simulink model "c00010M_harness"  (R2018a)
settings: Solver=FixedStepAuto  StartTime=0.0  StopTime=300  FixedStep=0.1  RelTol=1e-3
undefined symbols (not defined in the file): A1, hmax, PriorityTank, R1, R2, sigbuilder_block, TempThreshold
(part 29 of 40)

== system c00010M_harness/M119/Tank2/Control/ManualControlLiquidInOut ==
  Fill : Inport
  Empty : Inport  Port=2
  LiquidLevel : Inport  Port=3
  Constant : Constant  Value=hmax*0.9
  Constant1 : Constant  Value=0.9
  Logical Operator{,1..2,4} (4 alike) : Logic  AllPortsSameDT=off  OutDataTypeStr=boolean
  Logical Operator3 : Logic  Operator=NOT  AllPortsSameDT=off  OutDataTypeStr=boolean
  Logical Operator5 : Logic  Operator=NOT  AllPortsSameDT=off  OutDataTypeStr=boolean
  Relational Operator1 : RelationalOperator  Operator=<  OutDataTypeStr=boolean  RndMeth=Simplest
  Relational Operator2 : RelationalOperator  Operator=<  OutDataTypeStr=boolean  RndMeth=Simplest
  LiquidIn : Outport
  LiquidOut : Outport  Port=2
  wires:
  Empty/1 -> Logical Operator1/2
  Constant/1 -> Relational Operator1/2
  Relational Operator1/1 -> Logical Operator/2
  Fill/1 -> Logical Operator/1
  Logical Operator/1 -> Logical Operator5/1, Logical Operator2/1
  Relational Operator2/1 -> Logical Operator1/1
  Logical Operator1/1 -> Logical Operator3/1, Logical Operator4/2
  Constant1/1 -> Relational Operator2/1
  LiquidLevel/1 -> Relational Operator2/2, Relational Operator1/1
  Logical Operator3/1 -> Logical Operator2/2
  Logical Operator2/1 -> LiquidIn/1
  Logical Operator5/1 -> Logical Operator4/1
  Logical Operator4/1 -> LiquidOut/1

== system c00010M_harness/M119/Tank3/Control/Maintenance ==
  Type : Inport
  StartMaintenance : Inport  Port=2
  LiquidLevel : Inport  Port=3
  Chart : Stateflow chart  TreatAsAtomicUnit=on
  LiquidIn : Outport
  LiquidOut : Outport  Port=2
  wires:
  StartMaintenance/1 -> Chart/2(StartMaintenance)
  Type/1 -> Chart/1(Type)
  LiquidLevel/1 -> Chart/3(LiquidLevel)
  Chart/1(LiquidIn) -> LiquidIn/1
  Chart/2(LiquidOut) -> LiquidOut/1

== system c00010M_harness/M119/Tank3/Control/ManualControlLiquidInOut ==
  Fill : Inport
  Empty : Inport  Port=2
  LiquidLevel : Inport  Port=3
  Constant : Constant  Value=hmax*0.9
  Constant1 : Constant  Value=0.001
  Logical Operator{,1..2,4} (4 alike) : Logic  AllPortsSameDT=off  OutDataTypeStr=boolean
  Logical Operator3 : Logic  Operator=NOT  AllPortsSameDT=off  OutDataTypeStr=boolean
  Logical Operator5 : Logic  Operator=NOT  AllPortsSameDT=off  OutDataTypeStr=boolean
  Relational Operator1 : RelationalOperator  Operator=<  OutDataTypeStr=boolean  RndMeth=Simplest
  Relational Operator2 : RelationalOperator  Operator=<  OutDataTypeStr=boolean  RndMeth=Simplest
  LiquidIn : Outport
  LiquidOut : Outport  Port=2
  wires:
  Empty/1 -> Logical Operator1/2
  Constant/1 -> Relational Operator1/2
  Relational Operator1/1 -> Logical Operator/2
  Fill/1 -> Logical Operator/1
  Logical Operator/1 -> Logical Operator5/1, Logical Operator2/1
  Relational Operator2/1 -> Logical Operator1/1
  Logical Operator1/1 -> Logical Operator3/1, Logical Operator4/2
  Constant1/1 -> Relational Operator2/1
  LiquidLevel/1 -> Relational Operator2/2, Relational Operator1/1
  Logical Operator3/1 -> Logical Operator2/2
  Logical Operator2/1 -> LiquidIn/1
  Logical Operator5/1 -> Logical Operator4/1
  Logical Operator4/1 -> LiquidOut/1

== system c00010M_harness/M119/Tank3/Control/ManualControlReference ==
  ManualReference : Inport
  LiquidLevel : Inport  Port=2
  Add : Sum  Inputs=+-
  Add1 : Sum  Inputs=+-
  Gain1 : Gain  Gain=0.95
  Gain2 : Gain  Gain=0.95
  Relational Operator : RelationalOperator  Operator=>  OutDataTypeStr=boolean  RndMeth=Simplest
  Relational Operator1 : RelationalOperator  Operator=<  OutDataTypeStr=boolean  RndMeth=Simplest
  Saturation1 : Saturate  UpperLimit=hmax*0.9  LowerLimit=0
  LiquidIn : Outport
  LiquidOut : Outport  Port=2
  wires:
  LiquidLevel/1 -> Relational Operator/2, Add/1, Add1/1, Gain2/1
  Relational Operator/1 -> LiquidIn/1
  Relational Operator1/1 -> LiquidOut/1
  Add/1 -> Add1/2
  Add1/1 -> Relational Operator1/2
  Gain1/1 -> Saturation1/1
  Gain2/1 -> Add/2
  ManualReference/1 -> Gain1/1
  Saturation1/1 -> Relational Operator1/1, Relational Operator/1

== system c00010M_harness/M120/Tank2/Control/ManualControlLiquidInOut ==
  Fill : Inport
  Empty : Inport  Port=2
  LiquidLevel : Inport  Port=3
  Constant : Constant  Value=hmax*0.9
  Constant1 : Constant  Value=0.001
  Logical Operator : Logic  Operator=OR  AllPortsSameDT=off  OutDataTypeStr=boolean
  Logical Operator1 : Logic  AllPortsSameDT=off  OutDataTypeStr=boolean
  Logical Operator2 : Logic  AllPortsSameDT=off  OutDataTypeStr=boolean
  Logical Operator3 : Logic  Operator=NOT  AllPortsSameDT=off  OutDataTypeStr=boolean
  Logical Operator4 : Logic  AllPortsSameDT=off  OutDataTypeStr=boolean
  Logical Operator5 : Logic  Operator=NOT  AllPortsSameDT=off  OutDataTypeStr=boolean
  Relational Operator1 : RelationalOperator  Operator=<  OutDataTypeStr=boolean  RndMeth=Simplest
  Relational Operator2 : RelationalOperator  Operator=<  OutDataTypeStr=boolean  RndMeth=Simplest
  LiquidIn : Outport
  LiquidOut : Outport  Port=2
  wires:
  Empty/1 -> Logical Operator1/2
  Constant/1 -> Relational Operator1/2
  Relational Operator1/1 -> Logical Operator/2
  Fill/1 -> Logical Operator/1
  Logical Operator/1 -> Logical Operator5/1, Logical Operator2/1
  Relational Operator2/1 -> Logical Operator1/1
  Logical Operator1/1 -> Logical Operator3/1, Logical Operator4/2
  Constant1/1 -> Relational Operator2/1
  LiquidLevel/1 -> Relational Operator2/2, Relational Operator1/1
  Logical Operator3/1 -> Logical Operator2/2
  Logical Operator2/1 -> LiquidIn/1
  Logical Operator5/1 -> Logical Operator4/1
  Logical Operator4/1 -> LiquidOut/1

== system c00010M_harness/M120/Tank3/Control/Maintenance ==
  Type : Inport
  StartMaintenance : Inport  Port=2
  LiquidLevel : Inport  Port=3
  Chart : Stateflow chart  TreatAsAtomicUnit=on
  LiquidIn : Outport
  LiquidOut : Outport  Port=2
  wires:
  StartMaintenance/1 -> Chart/2(StartMaintenance)
  Type/1 -> Chart/1(Type)
  LiquidLevel/1 -> Chart/3(LiquidLevel)
  Chart/1(LiquidIn) -> LiquidIn/1
  Chart/2(LiquidOut) -> LiquidOut/1

== system c00010M_harness/M120/Tank3/Control/ManualControlLiquidInOut ==
  Fill : Inport
  Empty : Inport  Port=2
  LiquidLevel : Inport  Port=3
  Constant : Constant  Value=hmax*0.9
  Constant1 : Constant  Value=0.001
  Logical Operator{,1..2,4} (4 alike) : Logic  AllPortsSameDT=off  OutDataTypeStr=boolean
  Logical Operator3 : Logic  Operator=NOT  AllPortsSameDT=off  OutDataTypeStr=boolean
  Logical Operator5 : Logic  Operator=NOT  AllPortsSameDT=off  OutDataTypeStr=boolean
  Relational Operator1 : RelationalOperator  Operator=<  OutDataTypeStr=boolean  RndMeth=Simplest
  Relational Operator2 : RelationalOperator  Operator=<  OutDataTypeStr=boolean  RndMeth=Simplest
  LiquidIn : Outport
  LiquidOut : Outport  Port=2
  wires:
  Empty/1 -> Logical Operator1/2
  Constant/1 -> Relational Operator1/2
  Relational Operator1/1 -> Logical Operator/2
  Fill/1 -> Logical Operator/1
  Logical Operator/1 -> Logical Operator5/1, Logical Operator2/1
  Relational Operator2/1 -> Logical Operator1/1
  Logical Operator1/1 -> Logical Operator3/1, Logical Operator4/2
  Constant1/1 -> Relational Operator2/1
  LiquidLevel/1 -> Relational Operator2/2, Relational Operator1/1
  Logical Operator3/1 -> Logical Operator2/2
  Logical Operator2/1 -> LiquidIn/1
  Logical Operator5/1 -> Logical Operator4/1
  Logical Operator4/1 -> LiquidOut/1

== system c00010M_harness/M120/Tank3/Control/ManualControlReference ==
  ManualReference : Inport
  LiquidLevel : Inport  Port=2
  Add : Sum  Inputs=+-
  Add1 : Sum  Inputs=+-
  Gain1 : Gain  Gain=0.95
  Gain2 : Gain  Gain=0.95
  Relational Operator : RelationalOperator  Operator=>  OutDataTypeStr=boolean  RndMeth=Simplest
  Relational Operator1 : RelationalOperator  Operator=<  OutDataTypeStr=boolean  RndMeth=Simplest
  Saturation1 : Saturate  UpperLimit=hmax*0.9  LowerLimit=0
  LiquidIn : Outport
  LiquidOut : Outport  Port=2
  wires:
  LiquidLevel/1 -> Relational Operator/2, Add/1, Add1/1, Gain2/1
  Relational Operator/1 -> LiquidIn/1
  Relational Operator1/1 -> LiquidOut/1
  Add/1 -> Add1/2
  Add1/1 -> Relational Operator1/2
  Gain1/1 -> Saturation1/1
  Gain2/1 -> Add/2
  ManualReference/1 -> Gain1/1
  Saturation1/1 -> Relational Operator1/1, Relational Operator/1

== system c00010M_harness/M121/Tank2/Control/ManualControlLiquidInOut ==
  Fill : Inport
  Empty : Inport  Port=2
  LiquidLevel : Inport  Port=3
  Constant : Constant  Value=hmax*0.9
  Constant1 : Constant  Value=0.001
  Logical Operator : Logic  AllPortsSameDT=off  OutDataTypeStr=boolean
  Logical Operator1 : Logic  Operator=OR  AllPortsSameDT=off  OutDataTypeStr=boolean
  Logical Operator2 : Logic  AllPortsSameDT=off  OutDataTypeStr=boolean
  Logical Operator3 : Logic  Operator=NOT  AllPortsSameDT=off  OutDataTypeStr=boolean
  Logical Operator4 : Logic  AllPortsSameDT=off  OutDataTypeStr=boolean
  Logical Operator5 : Logic  Operator=NOT  AllPortsSameDT=off  OutDataTypeStr=boolean
  Relational Operator1 : RelationalOperator  Operator=<  OutDataTypeStr=boolean  RndMeth=Simplest
  Relational Operator2 : RelationalOperator  Operator=<  OutDataTypeStr=boolean  RndMeth=Simplest
  LiquidIn : Outport
  LiquidOut : Outport  Port=2
  wires:
  Empty/1 -> Logical Operator1/2
  Constant/1 -> Relational Operator1/2
  Relational Operator1/1 -> Logical Operator/2
  Fill/1 -> Logical Operator/1
  Logical Operator/1 -> Logical Operator5/1, Logical Operator2/1
  Relational Operator2/1 -> Logical Operator1/1
  Logical Operator1/1 -> Logical Operator3/1, Logical Operator4/2
  Constant1/1 -> Relational Operator2/1
  LiquidLevel/1 -> Relational Operator2/2, Relational Operator1/1
  Logical Operator3/1 -> Logical Operator2/2
  Logical Operator2/1 -> LiquidIn/1
  Logical Operator5/1 -> Logical Operator4/1
  Logical Operator4/1 -> LiquidOut/1

== system c00010M_harness/M121/Tank3/Control/Maintenance ==
  Type : Inport
  StartMaintenance : Inport  Port=2
  LiquidLevel : Inport  Port=3
  Chart : Stateflow chart  TreatAsAtomicUnit=on
  LiquidIn : Outport
  LiquidOut : Outport  Port=2
  wires:
  StartMaintenance/1 -> Chart/2(StartMaintenance)
  Type/1 -> Chart/1(Type)
  LiquidLevel/1 -> Chart/3(LiquidLevel)
  Chart/1(LiquidIn) -> LiquidIn/1
  Chart/2(LiquidOut) -> LiquidOut/1

== system c00010M_harness/M121/Tank3/Control/ManualControlLiquidInOut ==
  Fill : Inport
  Empty : Inport  Port=2
  LiquidLevel : Inport  Port=3
  Constant : Constant  Value=hmax*0.9
  Constant1 : Constant  Value=0.001
  Logical Operator{,1..2,4} (4 alike) : Logic  AllPortsSameDT=off  OutDataTypeStr=boolean
  Logical Operator3 : Logic  Operator=NOT  AllPortsSameDT=off  OutDataTypeStr=boolean
  Logical Operator5 : Logic  Operator=NOT  AllPortsSameDT=off  OutDataTypeStr=boolean
  Relational Operator1 : RelationalOperator  Operator=<  OutDataTypeStr=boolean  RndMeth=Simplest
  Relational Operator2 : RelationalOperator  Operator=<  OutDataTypeStr=boolean  RndMeth=Simplest
  LiquidIn : Outport
  LiquidOut : Outport  Port=2
  wires:
  Empty/1 -> Logical Operator1/2
  Constant/1 -> Relational Operator1/2
  Relational Operator1/1 -> Logical Operator/2
  Fill/1 -> Logical Operator/1
  Logical Operator/1 -> Logical Operator5/1, Logical Operator2/1
  Relational Operator2/1 -> Logical Operator1/1
  Logical Operator1/1 -> Logical Operator3/1, Logical Operator4/2
  Constant1/1 -> Relational Operator2/1
  LiquidLevel/1 -> Relational Operator2/2, Relational Operator1/1
  Logical Operator3/1 -> Logical Operator2/2
  Logical Operator2/1 -> LiquidIn/1
  Logical Operator5/1 -> Logical Operator4/1
  Logical Operator4/1 -> LiquidOut/1

== system c00010M_harness/M121/Tank3/Control/ManualControlReference ==
  ManualReference : Inport
  LiquidLevel : Inport  Port=2
  Add : Sum  Inputs=+-
  Add1 : Sum  Inputs=+-
  Gain1 : Gain  Gain=0.95
  Gain2 : Gain  Gain=0.95
  Relational Operator : RelationalOperator  Operator=>  OutDataTypeStr=boolean  RndMeth=Simplest
  Relational Operator1 : RelationalOperator  Operator=<  OutDataTypeStr=boolean  RndMeth=Simplest
  Saturation1 : Saturate  UpperLimit=hmax*0.9  LowerLimit=0
  LiquidIn : Outport
  LiquidOut : Outport  Port=2
  wires:
  LiquidLevel/1 -> Relational Operator/2, Add/1, Add1/1, Gain2/1
  Relational Operator/1 -> LiquidIn/1
  Relational Operator1/1 -> LiquidOut/1
  Add/1 -> Add1/2
  Add1/1 -> Relational Operator1/2
  Gain1/1 -> Saturation1/1
  Gain2/1 -> Add/2
  ManualReference/1 -> Gain1/1
  Saturation1/1 -> Relational Operator1/1, Relational Operator/1

== system c00010M_harness/M122/Tank2/Control/ManualControlLiquidInOut ==
  Fill : Inport
  Empty : Inport  Port=2
  LiquidLevel : Inport  Port=3
  Constant : Constant  Value=hmax*0.9
  Constant1 : Constant  Value=0.001
  Logical Operator : Logic  AllPortsSameDT=off  OutDataTypeStr=boolean
  Logical Operator1 : Logic  AllPortsSameDT=off  OutDataTypeStr=boolean
  Logical Operator2 : Logic  Operator=OR  AllPortsSameDT=off  OutDataTypeStr=boolean
  Logical Operator3 : Logic  Operator=NOT  AllPortsSameDT=off  OutDataTypeStr=boolean
  Logical Operator4 : Logic  AllPortsSameDT=off  OutDataTypeStr=boolean
  Logical Operator5 : Logic  Operator=NOT  AllPortsSameDT=off  OutDataTypeStr=boolean
  Relational Operator1 : RelationalOperator  Operator=<  OutDataTypeStr=boolean  RndMeth=Simplest
  Relational Operator2 : RelationalOperator  Operator=<  OutDataTypeStr=boolean  RndMeth=Simplest
  LiquidIn : Outport
  LiquidOut : Outport  Port=2
  wires:
  Empty/1 -> Logical Operator1/2
  Constant/1 -> Relational Operator1/2
  Relational Operator1/1 -> Logical Operator/2
  Fill/1 -> Logical Operator/1
  Logical Operator/1 -> Logical Operator5/1, Logical Operator2/1
  Relational Operator2/1 -> Logical Operator1/1
  Logical Operator1/1 -> Logical Operator3/1, Logical Operator4/2
  Constant1/1 -> Relational Operator2/1
  LiquidLevel/1 -> Relational Operator2/2, Relational Operator1/1
  Logical Operator3/1 -> Logical Operator2/2
  Logical Operator2/1 -> LiquidIn/1
  Logical Operator5/1 -> Logical Operator4/1
  Logical Operator4/1 -> LiquidOut/1

== system c00010M_harness/M122/Tank3/Control/Maintenance ==
  Type : Inport
  StartMaintenance : Inport  Port=2
  LiquidLevel : Inport  Port=3
  Chart : Stateflow chart  TreatAsAtomicUnit=on
  LiquidIn : Outport
  LiquidOut : Outport  Port=2
  wires:
  StartMaintenance/1 -> Chart/2(StartMaintenance)
  Type/1 -> Chart/1(Type)
  LiquidLevel/1 -> Chart/3(LiquidLevel)
  Chart/1(LiquidIn) -> LiquidIn/1
  Chart/2(LiquidOut) -> LiquidOut/1

== system c00010M_harness/M122/Tank3/Control/ManualControlLiquidInOut ==
  Fill : Inport
  Empty : Inport  Port=2
  LiquidLevel : Inport  Port=3
  Constant : Constant  Value=hmax*0.9
  Constant1 : Constant  Value=0.001
  Logical Operator{,1..2,4} (4 alike) : Logic  AllPortsSameDT=off  OutDataTypeStr=boolean
  Logical Operator3 : Logic  Operator=NOT  AllPortsSameDT=off  OutDataTypeStr=boolean
  Logical Operator5 : Logic  Operator=NOT  AllPortsSameDT=off  OutDataTypeStr=boolean
  Relational Operator1 : RelationalOperator  Operator=<  OutDataTypeStr=boolean  RndMeth=Simplest
  Relational Operator2 : RelationalOperator  Operator=<  OutDataTypeStr=boolean  RndMeth=Simplest
  LiquidIn : Outport
  LiquidOut : Outport  Port=2
  wires:
  Empty/1 -> Logical Operator1/2
  Constant/1 -> Relational Operator1/2
  Relational Operator1/1 -> Logical Operator/2
  Fill/1 -> Logical Operator/1
  Logical Operator/1 -> Logical Operator5/1, Logical Operator2/1
  Relational Operator2/1 -> Logical Operator1/1
  Logical Operator1/1 -> Logical Operator3/1, Logical Operator4/2
  Constant1/1 -> Relational Operator2/1
  LiquidLevel/1 -> Relational Operator2/2, Relational Operator1/1
  Logical Operator3/1 -> Logical Operator2/2
  Logical Operator2/1 -> LiquidIn/1
  Logical Operator5/1 -> Logical Operator4/1
  Logical Operator4/1 -> LiquidOut/1

== system c00010M_harness/M122/Tank3/Control/ManualControlReference ==
  ManualReference : Inport
  LiquidLevel : Inport  Port=2
  Add : Sum  Inputs=+-
  Add1 : Sum  Inputs=+-
  Gain1 : Gain  Gain=0.95
  Gain2 : Gain  Gain=0.95
  Relational Operator : RelationalOperator  Operator=>  OutDataTypeStr=boolean  RndMeth=Simplest
  Relational Operator1 : RelationalOperator  Operator=<  OutDataTypeStr=boolean  RndMeth=Simplest
  Saturation1 : Saturate  UpperLimit=hmax*0.9  LowerLimit=0
  LiquidIn : Outport
  LiquidOut : Outport  Port=2
  wires:
  LiquidLevel/1 -> Relational Operator/2, Add/1, Add1/1, Gain2/1
  Relational Operator/1 -> LiquidIn/1
  Relational Operator1/1 -> LiquidOut/1
  Add/1 -> Add1/2
  Add1/1 -> Relational Operator1/2
  Gain1/1 -> Saturation1/1
  Gain2/1 -> Add/2
  ManualReference/1 -> Gain1/1
  Saturation1/1 -> Relational Operator1/1, Relational Operator/1

== system c00010M_harness/M123/Tank2/Control/ManualControlLiquidInOut ==
  Fill : Inport
  Empty : Inport  Port=2
  LiquidLevel : Inport  Port=3
  Constant : Constant  Value=hmax*0.9
  Constant1 : Constant  Value=0.001
  Logical Operator{,1..2,4} (4 alike) : Logic  AllPortsSameDT=off  OutDataTypeStr=boolean
  Logical Operator5 : Logic  Operator=NOT  AllPortsSameDT=off  OutDataTypeStr=boolean
  Relational Operator1 : RelationalOperator  Operator=<  OutDataTypeStr=boolean  RndMeth=Simplest
  Relational Operator2 : RelationalOperator  Operator=<  OutDataTypeStr=boolean  RndMeth=Simplest
  LiquidIn : Outport
  LiquidOut : Outport  Port=2
  wires:
  Empty/1 -> Logical Operator1/2
  Constant/1 -> Relational Operator1/2
  Relational Operator1/1 -> Logical Operator/2
  Fill/1 -> Logical Operator/1
  Logical Operator/1 -> Logical Operator5/1, Logical Operator2/1
  Relational Operator2/1 -> Logical Operator1/1
  Constant1/1 -> Relational Operator2/1
  LiquidLevel/1 -> Relational Operator2/2, Relational Operator1/1
  Logical Operator1/1 -> Logical Operator2/2, Logical Operator4/2
  Logical Operator2/1 -> LiquidIn/1
  Logical Operator5/1 -> Logical Operator4/1
  Logical Operator4/1 -> LiquidOut/1

== system c00010M_harness/M123/Tank3/Control/Maintenance ==
  Type : Inport
  StartMaintenance : Inport  Port=2
  LiquidLevel : Inport  Port=3
  Chart : Stateflow chart  TreatAsAtomicUnit=on
  LiquidIn : Outport
  LiquidOut : Outport  Port=2
  wires:
  StartMaintenance/1 -> Chart/2(StartMaintenance)
  Type/1 -> Chart/1(Type)
  LiquidLevel/1 -> Chart/3(LiquidLevel)
  Chart/1(LiquidIn) -> LiquidIn/1
  Chart/2(LiquidOut) -> LiquidOut/1

== system c00010M_harness/M123/Tank3/Control/ManualControlLiquidInOut ==
  Fill : Inport
  Empty : Inport  Port=2
  LiquidLevel : Inport  Port=3
  Constant : Constant  Value=hmax*0.9
  Constant1 : Constant  Value=0.001
  Logical Operator{,1..2,4} (4 alike) : Logic  AllPortsSameDT=off  OutDataTypeStr=boolean
  Logical Operator3 : Logic  Operator=NOT  AllPortsSameDT=off  OutDataTypeStr=boolean
  Logical Operator5 : Logic  Operator=NOT  AllPortsSameDT=off  OutDataTypeStr=boolean
  Relational Operator1 : RelationalOperator  Operator=<  OutDataTypeStr=boolean  RndMeth=Simplest
  Relational Operator2 : RelationalOperator  Operator=<  OutDataTypeStr=boolean  RndMeth=Simplest
  LiquidIn : Outport
  LiquidOut : Outport  Port=2
  wires:
  Empty/1 -> Logical Operator1/2
  Constant/1 -> Relational Operator1/2
  Relational Operator1/1 -> Logical Operator/2
  Fill/1 -> Logical Operator/1
  Logical Operator/1 -> Logical Operator5/1, Logical Operator2/1
  Relational Operator2/1 -> Logical Operator1/1
  Logical Operator1/1 -> Logical Operator3/1, Logical Operator4/2
  Constant1/1 -> Relational Operator2/1
  LiquidLevel/1 -> Relational Operator2/2, Relational Operator1/1
  Logical Operator3/1 -> Logical Operator2/2
  Logical Operator2/1 -> LiquidIn/1
  Logical Operator5/1 -> Logical Operator4/1
  Logical Operator4/1 -> LiquidOut/1

== system c00010M_harness/M123/Tank3/Control/ManualControlReference ==
  ManualReference : Inport
  LiquidLevel : Inport  Port=2
  Add : Sum  Inputs=+-
  Add1 : Sum  Inputs=+-
  Gain1 : Gain  Gain=0.95
  Gain2 : Gain  Gain=0.95
  Relational Operator : RelationalOperator  Operator=>  OutDataTypeStr=boolean  RndMeth=Simplest
  Relational Operator1 : RelationalOperator  Operator=<  OutDataTypeStr=boolean  RndMeth=Simplest
  Saturation1 : Saturate  UpperLimit=hmax*0.9  LowerLimit=0
  LiquidIn : Outport
  LiquidOut : Outport  Port=2
  wires:
  LiquidLevel/1 -> Relational Operator/2, Add/1, Add1/1, Gain2/1
  Relational Operator/1 -> LiquidIn/1
  Relational Operator1/1 -> LiquidOut/1
  Add/1 -> Add1/2
  Add1/1 -> Relational Operator1/2
  Gain1/1 -> Saturation1/1
  Gain2/1 -> Add/2
  ManualReference/1 -> Gain1/1
  Saturation1/1 -> Relational Operator1/1, Relational Operator/1

== system c00010M_harness/M124/Tank2/Control/ManualControlLiquidInOut ==
  Fill : Inport
  Empty : Inport  Port=2
  LiquidLevel : Inport  Port=3
  Constant : Constant  Value=hmax*0.9
  Constant1 : Constant  Value=0.001
  Logical Operator : Logic  AllPortsSameDT=off  OutDataTypeStr=boolean
  Logical Operator1 : Logic  AllPortsSameDT=off  OutDataTypeStr=boolean
  Logical Operator2 : Logic  AllPortsSameDT=off  OutDataTypeStr=boolean
  Logical Operator3 : Logic  Operator=NOT  AllPortsSameDT=off  OutDataTypeStr=boolean
  Logical Operator4 : Logic  Operator=OR  AllPortsSameDT=off  OutDataTypeStr=boolean
  Logical Operator5 : Logic  Operator=NOT  AllPortsSameDT=off  OutDataTypeStr=boolean
  Relational Operator1 : RelationalOperator  Operator=<  OutDataTypeStr=boolean  RndMeth=Simplest
  Relational Operator2 : RelationalOperator  Operator=<  OutDataTypeStr=boolean  RndMeth=Simplest
  LiquidIn : Outport
  LiquidOut : Outport  Port=2
  wires:
  Empty/1 -> Logical Operator1/2
  Constant/1 -> Relational Operator1/2
  Relational Operator1/1 -> Logical Operator/2
  Fill/1 -> Logical Operator/1
  Logical Operator/1 -> Logical Operator5/1, Logical Operator2/1
  Relational Operator2/1 -> Logical Operator1/1
  Logical Operator1/1 -> Logical Operator3/1, Logical Operator4/2
  Constant1/1 -> Relational Operator2/1
  LiquidLevel/1 -> Relational Operator2/2, Relational Operator1/1
  Logical Operator3/1 -> Logical Operator2/2
  Logical Operator2/1 -> LiquidIn/1
  Logical Operator5/1 -> Logical Operator4/1
  Logical Operator4/1 -> LiquidOut/1

== system c00010M_harness/M124/Tank3/Control/Maintenance ==
  Type : Inport
  StartMaintenance : Inport  Port=2
  LiquidLevel : Inport  Port=3
  Chart : Stateflow chart  TreatAsAtomicUnit=on
  LiquidIn : Outport
  LiquidOut : Outport  Port=2
  wires:
  StartMaintenance/1 -> Chart/2(StartMaintenance)
  Type/1 -> Chart/1(Type)
  LiquidLevel/1 -> Chart/3(LiquidLevel)
  Chart/1(LiquidIn) -> LiquidIn/1
  Chart/2(LiquidOut) -> LiquidOut/1

== system c00010M_harness/M124/Tank3/Control/ManualControlLiquidInOut ==
  Fill : Inport
  Empty : Inport  Port=2
  LiquidLevel : Inport  Port=3
  Constant : Constant  Value=hmax*0.9
  Constant1 : Constant  Value=0.001
  Logical Operator{,1..2,4} (4 alike) : Logic  AllPortsSameDT=off  OutDataTypeStr=boolean
  Logical Operator3 : Logic  Operator=NOT  AllPortsSameDT=off  OutDataTypeStr=boolean
  Logical Operator5 : Logic  Operator=NOT  AllPortsSameDT=off  OutDataTypeStr=boolean
  Relational Operator1 : RelationalOperator  Operator=<  OutDataTypeStr=boolean  RndMeth=Simplest
  Relational Operator2 : RelationalOperator  Operator=<  OutDataTypeStr=boolean  RndMeth=Simplest
  LiquidIn : Outport
  LiquidOut : Outport  Port=2
  wires:
  Empty/1 -> Logical Operator1/2
  Constant/1 -> Relational Operator1/2
  Relational Operator1/1 -> Logical Operator/2
  Fill/1 -> Logical Operator/1
  Logical Operator/1 -> Logical Operator5/1, Logical Operator2/1
  Relational Operator2/1 -> Logical Operator1/1
  Logical Operator1/1 -> Logical Operator3/1, Logical Operator4/2
  Constant1/1 -> Relational Operator2/1
  LiquidLevel/1 -> Relational Operator2/2, Relational Operator1/1
  Logical Operator3/1 -> Logical Operator2/2
  Logical Operator2/1 -> LiquidIn/1
  Logical Operator5/1 -> Logical Operator4/1
  Logical Operator4/1 -> LiquidOut/1

== system c00010M_harness/M124/Tank3/Control/ManualControlReference ==
  ManualReference : Inport
  LiquidLevel : Inport  Port=2
  Add : Sum  Inputs=+-
  Add1 : Sum  Inputs=+-
  Gain1 : Gain  Gain=0.95
  Gain2 : Gain  Gain=0.95
  Relational Operator : RelationalOperator  Operator=>  OutDataTypeStr=boolean  RndMeth=Simplest
  Relational Operator1 : RelationalOperator  Operator=<  OutDataTypeStr=boolean  RndMeth=Simplest
  Saturation1 : Saturate  UpperLimit=hmax*0.9  LowerLimit=0
  LiquidIn : Outport
  LiquidOut : Outport  Port=2
  wires:
  LiquidLevel/1 -> Relational Operator/2, Add/1, Add1/1, Gain2/1
  Relational Operator/1 -> LiquidIn/1
  Relational Operator1/1 -> LiquidOut/1
  Add/1 -> Add1/2
  Add1/1 -> Relational Operator1/2
  Gain1/1 -> Saturation1/1
  Gain2/1 -> Add/2
  ManualReference/1 -> Gain1/1
  Saturation1/1 -> Relational Operator1/1, Relational Operator/1

== system c00010M_harness/M125/Tank2/Control/ManualControlLiquidInOut ==
  Fill : Inport
  Empty : Inport  Port=2
  LiquidLevel : Inport  Port=3
  Constant : Constant  Value=hmax*0.9
  Constant1 : Constant  Value=0.001
  Logical Operator{,1..2,4} (4 alike) : Logic  AllPortsSameDT=off  OutDataTypeStr=boolean
  Logical Operator3 : Logic  Operator=NOT  AllPortsSameDT=off  OutDataTypeStr=boolean
  Relational Operator1 : RelationalOperator  Operator=<  OutDataTypeStr=boolean  RndMeth=Simplest
  Relational Operator2 : RelationalOperator  Operator=<  OutDataTypeStr=boolean  RndMeth=Simplest
  LiquidIn : Outport
  LiquidOut : Outport  Port=2
  wires:
  Empty/1 -> Logical Operator1/2
  Constant/1 -> Relational Operator1/2
  Relational Operator1/1 -> Logical Operator/2
  Fill/1 -> Logical Operator/1
  Relational Operator2/1 -> Logical Operator1/1
  Logical Operator1/1 -> Logical Operator3/1, Logical Operator4/2
  Constant1/1 -> Relational Operator2/1
  LiquidLevel/1 -> Relational Operator2/2, Relational Operator1/1
  Logical Operator3/1 -> Logical Operator2/2
  Logical Operator2/1 -> LiquidIn/1
  Logical Operator/1 -> Logical Operator4/1, Logical Operator2/1
  Logical Operator4/1 -> LiquidOut/1

== system c00010M_harness/M125/Tank3/Control/Maintenance ==
  Type : Inport
  StartMaintenance : Inport  Port=2
  LiquidLevel : Inport  Port=3
  Chart : Stateflow chart  TreatAsAtomicUnit=on
  LiquidIn : Outport
  LiquidOut : Outport  Port=2
  wires:
  StartMaintenance/1 -> Chart/2(StartMaintenance)
  Type/1 -> Chart/1(Type)
  LiquidLevel/1 -> Chart/3(LiquidLevel)
  Chart/1(LiquidIn) -> LiquidIn/1
  Chart/2(LiquidOut) -> LiquidOut/1

== system c00010M_harness/M125/Tank3/Control/ManualControlLiquidInOut ==
  Fill : Inport
  Empty : Inport  Port=2
  LiquidLevel : Inport  Port=3
  Constant : Constant  Value=hmax*0.9
  Constant1 : Constant  Value=0.001
  Logical Operator{,1..2,4} (4 alike) : Logic  AllPortsSameDT=off  OutDataTypeStr=boolean
  Logical Operator3 : Logic  Operator=NOT  AllPortsSameDT=off  OutDataTypeStr=boolean
  Logical Operator5 : Logic  Operator=NOT  AllPortsSameDT=off  OutDataTypeStr=boolean
  Relational Operator1 : RelationalOperator  Operator=<  OutDataTypeStr=boolean  RndMeth=Simplest
  Relational Operator2 : RelationalOperator  Operator=<  OutDataTypeStr=boolean  RndMeth=Simplest
  LiquidIn : Outport
  LiquidOut : Outport  Port=2
  wires:
  Empty/1 -> Logical Operator1/2
  Constant/1 -> Relational Operator1/2
  Relational Operator1/1 -> Logical Operator/2
  Fill/1 -> Logical Operator/1
  Logical Operator/1 -> Logical Operator5/1, Logical Operator2/1
  Relational Operator2/1 -> Logical Operator1/1
  Logical Operator1/1 -> Logical Operator3/1, Logical Operator4/2
  Constant1/1 -> Relational Operator2/1
  LiquidLevel/1 -> Relational Operator2/2, Relational Operator1/1
  Logical Operator3/1 -> Logical Operator2/2
  Logical Operator2/1 -> LiquidIn/1
  Logical Operator5/1 -> Logical Operator4/1
  Logical Operator4/1 -> LiquidOut/1

== system c00010M_harness/M125/Tank3/Control/ManualControlReference ==
  ManualReference : Inport
  LiquidLevel : Inport  Port=2
  Add : Sum  Inputs=+-
  Add1 : Sum  Inputs=+-
  Gain1 : Gain  Gain=0.95
  Gain2 : Gain  Gain=0.95
  Relational Operator : RelationalOperator  Operator=>  OutDataTypeStr=boolean  RndMeth=Simplest
  Relational Operator1 : RelationalOperator  Operator=<  OutDataTypeStr=boolean  RndMeth=Simplest
  Saturation1 : Saturate  UpperLimit=hmax*0.9  LowerLimit=0
  LiquidIn : Outport
  LiquidOut : Outport  Port=2
  wires:
  LiquidLevel/1 -> Relational Operator/2, Add/1, Add1/1, Gain2/1
  Relational Operator/1 -> LiquidIn/1
  Relational Operator1/1 -> LiquidOut/1
  Add/1 -> Add1/2
  Add1/1 -> Relational Operator1/2
  Gain1/1 -> Saturation1/1
  Gain2/1 -> Add/2
  ManualReference/1 -> Gain1/1
  Saturation1/1 -> Relational Operator1/1, Relational Operator/1

== system c00010M_harness/M126/Tank2/Control/ManualControlLiquidInOut ==
  Fill : Inport
  Empty : Inport  Port=2
  LiquidLevel : Inport  Port=3
  Constant : Constant  Value=hmax*0.9
  Constant1 : Constant  Value=0.001
  Logical Operator{,1..2,4} (4 alike) : Logic  AllPortsSameDT=off  OutDataTypeStr=boolean
  Logical Operator3 : Logic  Operator=NOT  AllPortsSameDT=off  OutDataTypeStr=boolean
  Logical Operator5 : Logic  Operator=NOT  AllPortsSameDT=off  OutDataTypeStr=boolean
  Relational Operator1 : RelationalOperator  Operator=>  OutDataTypeStr=boolean  RndMeth=Simplest
  Relational Operator2 : RelationalOperator  Operator=<  OutDataTypeStr=boolean  RndMeth=Simplest
  LiquidIn : Outport
  LiquidOut : Outport  Port=2
  wires:
  Empty/1 -> Logical Operator1/2
  Constant/1 -> Relational Operator1/2
  Relational Operator1/1 -> Logical Operator/2
  Fill/1 -> Logical Operator/1
  Logical Operator/1 -> Logical Operator5/1, Logical Operator2/1
  Relational Operator2/1 -> Logical Operator1/1
  Logical Operator1/1 -> Logical Operator3/1, Logical Operator4/2
  Constant1/1 -> Relational Operator2/1
  LiquidLevel/1 -> Relational Operator2/2, Relational Operator1/1
  Logical Operator3/1 -> Logical Operator2/2
  Logical Operator2/1 -> LiquidIn/1
  Logical Operator5/1 -> Logical Operator4/1
  Logical Operator4/1 -> LiquidOut/1

== system c00010M_harness/M126/Tank3/Control/Maintenance ==
  Type : Inport
  StartMaintenance : Inport  Port=2
  LiquidLevel : Inport  Port=3
  Chart : Stateflow chart  TreatAsAtomicUnit=on
  LiquidIn : Outport
  LiquidOut : Outport  Port=2
  wires:
  StartMaintenance/1 -> Chart/2(StartMaintenance)
  Type/1 -> Chart/1(Type)
  LiquidLevel/1 -> Chart/3(LiquidLevel)
  Chart/1(LiquidIn) -> LiquidIn/1
  Chart/2(LiquidOut) -> LiquidOut/1

== system c00010M_harness/M126/Tank3/Control/ManualControlLiquidInOut ==
  Fill : Inport
  Empty : Inport  Port=2
  LiquidLevel : Inport  Port=3
  Constant : Constant  Value=hmax*0.9
  Constant1 : Constant  Value=0.001
  Logical Operator{,1..2,4} (4 alike) : Logic  AllPortsSameDT=off  OutDataTypeStr=boolean
  Logical Operator3 : Logic  Operator=NOT  AllPortsSameDT=off  OutDataTypeStr=boolean
  Logical Operator5 : Logic  Operator=NOT  AllPortsSameDT=off  OutDataTypeStr=boolean
  Relational Operator1 : RelationalOperator  Operator=<  OutDataTypeStr=boolean  RndMeth=Simplest
  Relational Operator2 : RelationalOperator  Operator=<  OutDataTypeStr=boolean  RndMeth=Simplest
  LiquidIn : Outport
  LiquidOut : Outport  Port=2
  wires:
  Empty/1 -> Logical Operator1/2
  Constant/1 -> Relational Operator1/2
  Relational Operator1/1 -> Logical Operator/2
  Fill/1 -> Logical Operator/1
  Logical Operator/1 -> Logical Operator5/1, Logical Operator2/1
  Relational Operator2/1 -> Logical Operator1/1
  Logical Operator1/1 -> Logical Operator3/1, Logical Operator4/2
  Constant1/1 -> Relational Operator2/1
  LiquidLevel/1 -> Relational Operator2/2, Relational Operator1/1
  Logical Operator3/1 -> Logical Operator2/2
  Logical Operator2/1 -> LiquidIn/1
  Logical Operator5/1 -> Logical Operator4/1
  Logical Operator4/1 -> LiquidOut/1

== system c00010M_harness/M126/Tank3/Control/ManualControlReference ==
  ManualReference : Inport
  LiquidLevel : Inport  Port=2
  Add : Sum  Inputs=+-
  Add1 : Sum  Inputs=+-
  Gain1 : Gain  Gain=0.95
  Gain2 : Gain  Gain=0.95
  Relational Operator : RelationalOperator  Operator=>  OutDataTypeStr=boolean  RndMeth=Simplest
  Relational Operator1 : RelationalOperator  Operator=<  OutDataTypeStr=boolean  RndMeth=Simplest
  Saturation1 : Saturate  UpperLimit=hmax*0.9  LowerLimit=0
  LiquidIn : Outport
  LiquidOut : Outport  Port=2
  wires:
  LiquidLevel/1 -> Relational Operator/2, Add/1, Add1/1, Gain2/1
  Relational Operator/1 -> LiquidIn/1
  Relational Operator1/1 -> LiquidOut/1
  Add/1 -> Add1/2
  Add1/1 -> Relational Operator1/2
  Gain1/1 -> Saturation1/1
  Gain2/1 -> Add/2
  ManualReference/1 -> Gain1/1
  Saturation1/1 -> Relational Operator1/1, Relational Operator/1

== system c00010M_harness/M127/Tank2/Control/ManualControlLiquidInOut ==
  Fill : Inport
  Empty : Inport  Port=2
  LiquidLevel : Inport  Port=3
  Constant : Constant  Value=hmax*0.9
  Constant1 : Constant  Value=0.001
  Logical Operator{,1..2,4} (4 alike) : Logic  AllPortsSameDT=off  OutDataTypeStr=boolean
  Logical Operator3 : Logic  Operator=NOT  AllPortsSameDT=off  OutDataTypeStr=boolean
  Logical Operator5 : Logic  Operator=NOT  AllPortsSameDT=off  OutDataTypeStr=boolean
  Relational Operator1 : RelationalOperator  Operator=<  OutDataTypeStr=boolean  RndMeth=Simplest
  Relational Operator2 : RelationalOperator  Operator=>  OutDataTypeStr=boolean  RndMeth=Simplest
  LiquidIn : Outport
  LiquidOut : Outport  Port=2
  wires:
  Empty/1 -> Logical Operator1/2
  Constant/1 -> Relational Operator1/2
  Relational Operator1/1 -> Logical Operator/2
  Fill/1 -> Logical Operator/1
  Logical Operator/1 -> Logical Operator5/1, Logical Operator2/1
  Relational Operator2/1 -> Logical Operator1/1
  Logical Operator1/1 -> Logical Operator3/1, Logical Operator4/2
  Constant1/1 -> Relational Operator2/1
  LiquidLevel/1 -> Relational Operator2/2, Relational Operator1/1
  Logical Operator3/1 -> Logical Operator2/2
  Logical Operator2/1 -> LiquidIn/1
  Logical Operator5/1 -> Logical Operator4/1
  Logical Operator4/1 -> LiquidOut/1

== system c00010M_harness/M127/Tank3/Control/Maintenance ==
  Type : Inport
  StartMaintenance : Inport  Port=2
  LiquidLevel : Inport  Port=3
  Chart : Stateflow chart  TreatAsAtomicUnit=on
  LiquidIn : Outport
  LiquidOut : Outport  Port=2
  wires:
  StartMaintenance/1 -> Chart/2(StartMaintenance)
  Type/1 -> Chart/1(Type)
  LiquidLevel/1 -> Chart/3(LiquidLevel)
  Chart/1(LiquidIn) -> LiquidIn/1
  Chart/2(LiquidOut) -> LiquidOut/1

== system c00010M_harness/M127/Tank3/Control/ManualControlLiquidInOut ==
  Fill : Inport
  Empty : Inport  Port=2
  LiquidLevel : Inport  Port=3
  Constant : Constant  Value=hmax*0.9
  Constant1 : Constant  Value=0.001
  Logical Operator{,1..2,4} (4 alike) : Logic  AllPortsSameDT=off  OutDataTypeStr=boolean
  Logical Operator3 : Logic  Operator=NOT  AllPortsSameDT=off  OutDataTypeStr=boolean
  Logical Operator5 : Logic  Operator=NOT  AllPortsSameDT=off  OutDataTypeStr=boolean
  Relational Operator1 : RelationalOperator  Operator=<  OutDataTypeStr=boolean  RndMeth=Simplest
  Relational Operator2 : RelationalOperator  Operator=<  OutDataTypeStr=boolean  RndMeth=Simplest
  LiquidIn : Outport
  LiquidOut : Outport  Port=2
  wires:
  Empty/1 -> Logical Operator1/2
  Constant/1 -> Relational Operator1/2
  Relational Operator1/1 -> Logical Operator/2
  Fill/1 -> Logical Operator/1
  Logical Operator/1 -> Logical Operator5/1, Logical Operator2/1
  Relational Operator2/1 -> Logical Operator1/1
  Logical Operator1/1 -> Logical Operator3/1, Logical Operator4/2
  Constant1/1 -> Relational Operator2/1
  LiquidLevel/1 -> Relational Operator2/2, Relational Operator1/1
  Logical Operator3/1 -> Logical Operator2/2
  Logical Operator2/1 -> LiquidIn/1
  Logical Operator5/1 -> Logical Operator4/1
  Logical Operator4/1 -> LiquidOut/1

== system c00010M_harness/M127/Tank3/Control/ManualControlReference ==
  ManualReference : Inport
  LiquidLevel : Inport  Port=2
  Add : Sum  Inputs=+-
  Add1 : Sum  Inputs=+-
  Gain1 : Gain  Gain=0.95
  Gain2 : Gain  Gain=0.95
  Relational Operator : RelationalOperator  Operator=>  OutDataTypeStr=boolean  RndMeth=Simplest
  Relational Operator1 : RelationalOperator  Operator=<  OutDataTypeStr=boolean  RndMeth=Simplest
  Saturation1 : Saturate  UpperLimit=hmax*0.9  LowerLimit=0
  LiquidIn : Outport
  LiquidOut : Outport  Port=2
  wires:
  LiquidLevel/1 -> Relational Operator/2, Add/1, Add1/1, Gain2/1
  Relational Operator/1 -> LiquidIn/1
  Relational Operator1/1 -> LiquidOut/1
  Add/1 -> Add1/2
  Add1/1 -> Relational Operator1/2
  Gain1/1 -> Saturation1/1
  Gain2/1 -> Add/2
  ManualReference/1 -> Gain1/1
  Saturation1/1 -> Relational Operator1/1, Relational Operator/1

== system c00010M_harness/M139/Tank2/Control/ManualControlLiquidInOut ==
  Fill : Inport
  Empty : Inport  Port=2
  LiquidLevel : Inport  Port=3
  Constant : Constant  Value=hmax*0.9
  Constant1 : Constant  Value=0.001
  Logical Operator{,1..2,4} (4 alike) : Logic  AllPortsSameDT=off  OutDataTypeStr=boolean
  Logical Operator3 : Logic  Operator=NOT  AllPortsSameDT=off  OutDataTypeStr=boolean
  Logical Operator5 : Logic  Operator=NOT  AllPortsSameDT=off  OutDataTypeStr=boolean
  Relational Operator1 : RelationalOperator  Operator=<  OutDataTypeStr=boolean  RndMeth=Simplest
  Relational Operator2 : RelationalOperator  Operator=<  OutDataTypeStr=boolean  RndMeth=Simplest
  LiquidIn : Outport
  LiquidOut : Outport  Port=2
  wires:
  Empty/1 -> Logical Operator1/2
  Constant/1 -> Relational Operator1/2
  Relational Operator1/1 -> Logical Operator/2
  Fill/1 -> Logical Operator/1
  Logical Operator/1 -> Logical Operator5/1, Logical Operator2/1
  Relational Operator2/1 -> Logical Operator1/1
  Logical Operator1/1 -> Logical Operator3/1, Logical Operator4/2
  Constant1/1 -> Relational Operator2/1
  LiquidLevel/1 -> Relational Operator2/2, Relational Operator1/1
  Logical Operator3/1 -> Logical Operator2/2
  Logical Operator2/1 -> LiquidIn/1
  Logical Operator5/1 -> Logical Operator4/1
  Logical Operator4/1 -> LiquidOut/1

== system c00010M_harness/M139/Tank3/Control/Maintenance ==
  Type : Inport
  StartMaintenance : Inport  Port=2
  LiquidLevel : Inport  Port=3
  Chart : Stateflow chart  TreatAsAtomicUnit=on
  LiquidIn : Outport
  LiquidOut : Outport  Port=2
  wires:
  StartMaintenance/1 -> Chart/2(StartMaintenance)
  Type/1 -> Chart/1(Type)
  LiquidLevel/1 -> Chart/3(LiquidLevel)
  Chart/1(LiquidIn) -> LiquidIn/1
  Chart/2(LiquidOut) -> LiquidOut/1

== system c00010M_harness/M139/Tank3/Control/ManualControlLiquidInOut ==
  Fill : Inport
  Empty : Inport  Port=2
  LiquidLevel : Inport  Port=3
  Constant : Constant  Value=hmax*0.9
  Constant1 : Constant  Value=0.001
  Logical Operator{,1..2,4} (4 alike) : Logic  AllPortsSameDT=off  OutDataTypeStr=boolean
  Logical Operator3 : Logic  Operator=NOT  AllPortsSameDT=off  OutDataTypeStr=boolean
  Logical Operator5 : Logic  Operator=NOT  AllPortsSameDT=off  OutDataTypeStr=boolean
  Relational Operator1 : RelationalOperator  Operator=<  OutDataTypeStr=boolean  RndMeth=Simplest
  Relational Operator2 : RelationalOperator  Operator=<  OutDataTypeStr=boolean  RndMeth=Simplest
  LiquidIn : Outport
  LiquidOut : Outport  Port=2
  wires:
  Empty/1 -> Logical Operator1/2
  Constant/1 -> Relational Operator1/2
  Relational Operator1/1 -> Logical Operator/2
  Fill/1 -> Logical Operator/1
  Logical Operator/1 -> Logical Operator5/1, Logical Operator2/1
  Relational Operator2/1 -> Logical Operator1/1
  Logical Operator1/1 -> Logical Operator3/1, Logical Operator4/2
  Constant1/1 -> Relational Operator2/1
  LiquidLevel/1 -> Relational Operator2/2, Relational Operator1/1
  Logical Operator3/1 -> Logical Operator2/2
  Logical Operator2/1 -> LiquidIn/1
  Logical Operator5/1 -> Logical Operator4/1
  Logical Operator4/1 -> LiquidOut/1

== system c00010M_harness/M139/Tank3/Control/ManualControlReference ==
  ManualReference : Inport
  LiquidLevel : Inport  Port=2
  Add : Sum  Inputs=+-
  Add1 : Sum  Inputs=+-
  Gain1 : Gain  Gain=0.95
  Gain2 : Gain  Gain=0.95
  Relational Operator : RelationalOperator  Operator=>  OutDataTypeStr=boolean  RndMeth=Simplest
  Relational Operator1 : RelationalOperator  Operator=<  OutDataTypeStr=boolean  RndMeth=Simplest
  Saturation1 : Saturate  UpperLimit=hmax*0.9  LowerLimit=0
  LiquidIn : Outport
  LiquidOut : Outport  Port=2
  wires:
  LiquidLevel/1 -> Relational Operator/2, Add/1, Add1/1, Gain2/1
  Relational Operator/1 -> LiquidIn/1
  Relational Operator1/1 -> LiquidOut/1
  Add/1 -> Add1/2
  Add1/1 -> Relational Operator1/2
  Gain1/1 -> Saturation1/1
  Gain2/1 -> Add/2
  ManualReference/1 -> Gain1/1
  Saturation1/1 -> Relational Operator1/1, Relational Operator/1

== system c00010M_harness/M140/Tank2/Control/ManualControlLiquidInOut ==
  Fill : Inport
  Empty : Inport  Port=2
  LiquidLevel : Inport  Port=3
  Constant : Constant  Value=hmax*0.9
  Constant1 : Constant  Value=0.001
  Logical Operator{,1..2,4} (4 alike) : Logic  AllPortsSameDT=off  OutDataTypeStr=boolean
  Logical Operator3 : Logic  Operator=NOT  AllPortsSameDT=off  OutDataTypeStr=boolean
  Logical Operator5 : Logic  Operator=NOT  AllPortsSameDT=off  OutDataTypeStr=boolean
  Relational Operator1 : RelationalOperator  Operator=<  OutDataTypeStr=boolean  RndMeth=Simplest
  Relational Operator2 : RelationalOperator  Operator=<  OutDataTypeStr=boolean  RndMeth=Simplest
  LiquidIn : Outport
  LiquidOut : Outport  Port=2
  wires:
  Empty/1 -> Logical Operator1/2
  Constant/1 -> Relational Operator1/2
  Relational Operator1/1 -> Logical Operator/2
  Fill/1 -> Logical Operator/1
  Logical Operator/1 -> Logical Operator5/1, Logical Operator2/1
  Relational Operator2/1 -> Logical Operator1/1
  Logical Operator1/1 -> Logical Operator3/1, Logical Operator4/2
  Constant1/1 -> Relational Operator2/1
  LiquidLevel/1 -> Relational Operator2/2, Relational Operator1/1
  Logical Operator3/1 -> Logical Operator2/2
  Logical Operator2/1 -> LiquidIn/1
  Logical Operator5/1 -> Logical Operator4/1
  Logical Operator4/1 -> LiquidOut/1

== system c00010M_harness/M140/Tank3/Control/Maintenance ==
  Type : Inport
  StartMaintenance : Inport  Port=2
  LiquidLevel : Inport  Port=3
  Chart : Stateflow chart  TreatAsAtomicUnit=on
  LiquidIn : Outport
  LiquidOut : Outport  Port=2
  wires:
  StartMaintenance/1 -> Chart/2(StartMaintenance)
  Type/1 -> Chart/1(Type)
  LiquidLevel/1 -> Chart/3(LiquidLevel)
  Chart/1(LiquidIn) -> LiquidIn/1
  Chart/2(LiquidOut) -> LiquidOut/1

== system c00010M_harness/M140/Tank3/Control/ManualControlLiquidInOut ==
  Fill : Inport
  Empty : Inport  Port=2
  LiquidLevel : Inport  Port=3
  Constant : Constant  Value=hmax*0.9
  Constant1 : Constant  Value=0.001
  Logical Operator{,1..2,4} (4 alike) : Logic  AllPortsSameDT=off  OutDataTypeStr=boolean
  Logical Operator3 : Logic  Operator=NOT  AllPortsSameDT=off  OutDataTypeStr=boolean
  Logical Operator5 : Logic  Operator=NOT  AllPortsSameDT=off  OutDataTypeStr=boolean
  Relational Operator1 : RelationalOperator  Operator=<  OutDataTypeStr=boolean  RndMeth=Simplest
  Relational Operator2 : RelationalOperator  Operator=<  OutDataTypeStr=boolean  RndMeth=Simplest
  LiquidIn : Outport
  LiquidOut : Outport  Port=2
  wires:
  Empty/1 -> Logical Operator1/2
  Constant/1 -> Relational Operator1/2
  Relational Operator1/1 -> Logical Operator/2
  Fill/1 -> Logical Operator/1
  Logical Operator/1 -> Logical Operator5/1, Logical Operator2/1
  Relational Operator2/1 -> Logical Operator1/1
  Logical Operator1/1 -> Logical Operator3/1, Logical Operator4/2
  Constant1/1 -> Relational Operator2/1
  LiquidLevel/1 -> Relational Operator2/2, Relational Operator1/1
  Logical Operator3/1 -> Logical Operator2/2
  Logical Operator2/1 -> LiquidIn/1
  Logical Operator5/1 -> Logical Operator4/1
  Logical Operator4/1 -> LiquidOut/1

== system c00010M_harness/M140/Tank3/Control/ManualControlReference ==
  ManualReference : Inport
  LiquidLevel : Inport  Port=2
  Add : Sum  Inputs=+-
  Add1 : Sum  Inputs=+-
  Gain1 : Gain  Gain=0.95
  Gain2 : Gain  Gain=0.95
  Relational Operator : RelationalOperator  Operator=>  OutDataTypeStr=boolean  RndMeth=Simplest
  Relational Operator1 : RelationalOperator  Operator=<  OutDataTypeStr=boolean  RndMeth=Simplest
  Saturation1 : Saturate  UpperLimit=hmax*0.9  LowerLimit=0
  LiquidIn : Outport
  LiquidOut : Outport  Port=2
  wires:
  LiquidLevel/1 -> Relational Operator/2, Add/1, Add1/1, Gain2/1
  Relational Operator/1 -> LiquidIn/1
  Relational Operator1/1 -> LiquidOut/1
  Add/1 -> Add1/2
  Add1/1 -> Relational Operator1/2
  Gain1/1 -> Saturation1/1
  Gain2/1 -> Add/2
  ManualReference/1 -> Gain1/1
  Saturation1/1 -> Relational Operator1/1, Relational Operator/1

== system c00010M_harness/M141/Tank2/Control/ManualControlLiquidInOut ==
  Fill : Inport
  Empty : Inport  Port=2
  LiquidLevel : Inport  Port=3
  Constant : Constant  Value=hmax*0.9
  Constant1 : Constant  Value=0.001
  Logical Operator{,1..2,4} (4 alike) : Logic  AllPortsSameDT=off  OutDataTypeStr=boolean
  Logical Operator3 : Logic  Operator=NOT  AllPortsSameDT=off  OutDataTypeStr=boolean
  Logical Operator5 : Logic  Operator=NOT  AllPortsSameDT=off  OutDataTypeStr=boolean
  Relational Operator1 : RelationalOperator  Operator=<  OutDataTypeStr=boolean  RndMeth=Simplest
  Relational Operator2 : RelationalOperator  Operator=<  OutDataTypeStr=boolean  RndMeth=Simplest
  LiquidIn : Outport
  LiquidOut : Outport  Port=2
  wires:
  Empty/1 -> Logical Operator1/2
  Constant/1 -> Relational Operator1/2
  Relational Operator1/1 -> Logical Operator/2
  Fill/1 -> Logical Operator/1
  Logical Operator/1 -> Logical Operator5/1, Logical Operator2/1
  Relational Operator2/1 -> Logical Operator1/1
  Logical Operator1/1 -> Logical Operator3/1, Logical Operator4/2
  Constant1/1 -> Relational Operator2/1
  LiquidLevel/1 -> Relational Operator2/2, Relational Operator1/1
  Logical Operator3/1 -> Logical Operator2/2
  Logical Operator2/1 -> LiquidIn/1
  Logical Operator5/1 -> Logical Operator4/1
  Logical Operator4/1 -> LiquidOut/1

== system c00010M_harness/M141/Tank3/Control/Maintenance ==
  Type : Inport
  StartMaintenance : Inport  Port=2
  LiquidLevel : Inport  Port=3
  Chart : Stateflow chart  TreatAsAtomicUnit=on
  LiquidIn : Outport
  LiquidOut : Outport  Port=2
  wires:
  StartMaintenance/1 -> Chart/2(StartMaintenance)
  Type/1 -> Chart/1(Type)
  LiquidLevel/1 -> Chart/3(LiquidLevel)
  Chart/1(LiquidIn) -> LiquidIn/1
  Chart/2(LiquidOut) -> LiquidOut/1

== system c00010M_harness/M141/Tank3/Control/ManualControlLiquidInOut ==
  Fill : Inport
  Empty : Inport  Port=2
  LiquidLevel : Inport  Port=3
  Constant : Constant  Value=hmax*0.9
  Constant1 : Constant  Value=0.001
  Logical Operator{,1..2,4} (4 alike) : Logic  AllPortsSameDT=off  OutDataTypeStr=boolean
  Logical Operator3 : Logic  Operator=NOT  AllPortsSameDT=off  OutDataTypeStr=boolean
  Logical Operator5 : Logic  Operator=NOT  AllPortsSameDT=off  OutDataTypeStr=boolean
  Relational Operator1 : RelationalOperator  Operator=<  OutDataTypeStr=boolean  RndMeth=Simplest
  Relational Operator2 : RelationalOperator  Operator=<  OutDataTypeStr=boolean  RndMeth=Simplest
  LiquidIn : Outport
  LiquidOut : Outport  Port=2
  wires:
  Empty/1 -> Logical Operator1/2
  Constant/1 -> Relational Operator1/2
  Relational Operator1/1 -> Logical Operator/2
  Fill/1 -> Logical Operator/1
  Logical Operator/1 -> Logical Operator5/1, Logical Operator2/1
  Relational Operator2/1 -> Logical Operator1/1
  Logical Operator1/1 -> Logical Operator3/1, Logical Operator4/2
  Constant1/1 -> Relational Operator2/1
  LiquidLevel/1 -> Relational Operator2/2, Relational Operator1/1
  Logical Operator3/1 -> Logical Operator2/2
  Logical Operator2/1 -> LiquidIn/1
  Logical Operator5/1 -> Logical Operator4/1
  Logical Operator4/1 -> LiquidOut/1

== system c00010M_harness/M141/Tank3/Control/ManualControlReference ==
  ManualReference : Inport
  LiquidLevel : Inport  Port=2
  Add : Sum  Inputs=+-
  Add1 : Sum  Inputs=+-
  Gain1 : Gain  Gain=0.95
  Gain2 : Gain  Gain=0.95
  Relational Operator : RelationalOperator  Operator=>  OutDataTypeStr=boolean  RndMeth=Simplest
  Relational Operator1 : RelationalOperator  Operator=<  OutDataTypeStr=boolean  RndMeth=Simplest
  Saturation1 : Saturate  UpperLimit=hmax*0.9  LowerLimit=0
  LiquidIn : Outport
  LiquidOut : Outport  Port=2
  wires:
  LiquidLevel/1 -> Relational Operator/2, Add/1, Add1/1, Gain2/1
  Relational Operator/1 -> LiquidIn/1
  Relational Operator1/1 -> LiquidOut/1
  Add/1 -> Add1/2
  Add1/1 -> Relational Operator1/2
  Gain1/1 -> Saturation1/1
  Gain2/1 -> Add/2
  ManualReference/1 -> Gain1/1
  Saturation1/1 -> Relational Operator1/1, Relational Operator/1
